simulink model "ThreePhasejojo"  (R2024a)
settings: Solver=VariableStepAuto  StartTime=0.0  StopTime=0.12  FixedStep=0.001s  MaxStep=0.00001  RelTol=1e-4
undefined symbols (not defined in the file): D1, Delta
libraries: spsVoltageMeasurementLib x19, spsCurrentMeasurementLib x12, spsPowerLib x10, spsACVoltageSourceLib x3, spsThreePhaseSeriesRLCBranchLib x3, spsGroundLib x3, spsSeriesRLCBranchLib x3, spsThreePhaseTransformerTwoWindingsLib x1, spsMutualInductanceLib x1, spspowerguiLib x1
settings Model: Creator=admin  LastModifiedBy=Asus

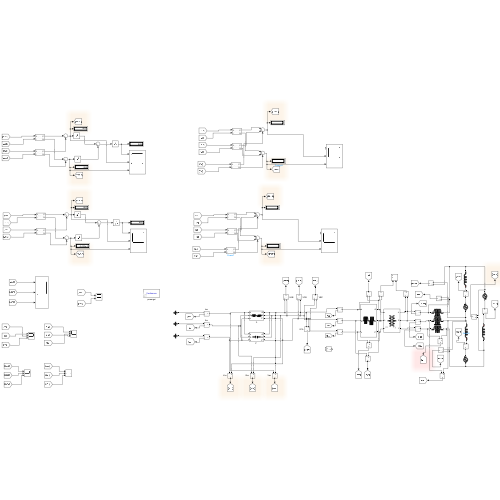
[thumbnail: Simulink's stored preview of the top-level diagram]
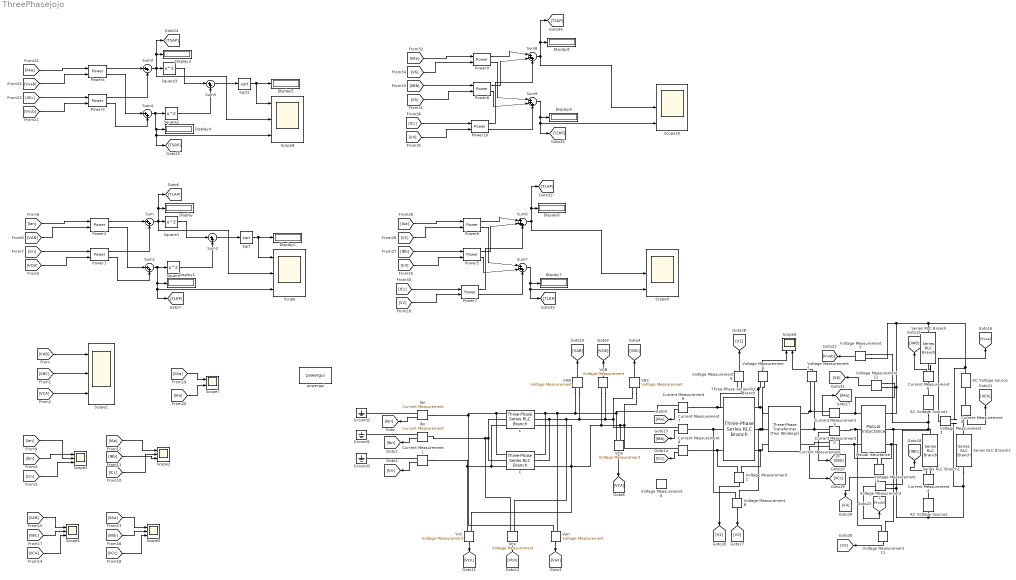
== system ThreePhasejojo ==
  " " : spsThreePhaseTransformerTwoWindingsLib/Three-Phase Transformer (Two Windings)  Winding1Connection=Yg  Winding2Connection=Delta (D1)  CoreType=Three single-phase transformers  SetSaturation=off  Hysteresis=off  DataFile='hysteresis'  SetInitialFlux=off  Measurements=None  UNITS=SI  NominalPower=[ 250e6 , 50 ]  Winding1=[380 1e-3 1e-3]  Winding2=[760 1e-3 1e-3]  Rm=1e3  Lm=1e3  L0=2.866  Saturation=[0 0;0.66653 1910.3;277.72 2419.7]  InitialFluxes=[1273.5 -1273.5 1114.3]  BreakLoop=off  DiscreteSolver=Trapezoidal iterative  DataType=on  TransfoNumber=1
  AC Voltage Source : spsACVoltageSourceLib/AC Voltage Source  Amplitude=380  Phase=-120  Frequency=50  SampleTime=0  Measurements=None  BusType=swing  Pref=10e3  Qref=0  Qmin=-inf  Qmax=+inf
  AC Voltage Source1 : spsACVoltageSourceLib/AC Voltage Source  Amplitude=380  Phase=0  Frequency=50  SampleTime=0  Measurements=None  BusType=swing  Pref=10e3  Qref=0  Qmin=-inf  Qmax=+inf
  AC Voltage Source2 : spsACVoltageSourceLib/AC Voltage Source  Amplitude=380  Phase=120  Frequency=50  SampleTime=0  Measurements=None  BusType=swing  Pref=10e3  Qref=0  Qmin=-inf  Qmax=+inf
  "C " : spsThreePhaseSeriesRLCBranchLib/Three-Phase Series RLC Branch  LConnTagsString=A|B|C  RConnTagsString=A|B|C  BranchType=C  Resistance=20  Inductance=0.1/pi  Capacitance=2e-4/pi  Measurements=None
  Current Measurement{1..10} (10 alike) : spsCurrentMeasurementLib/Current Measurement  PhasorSimulation=off  OutputType=Complex  PSBequivalent=0
  Display{,1..9} (10 alike) : Display
  Ground1 : spsGroundLib/Ground  LConnTagsString=a
  Ground2 : spsGroundLib/Ground  LConnTagsString=a
  Ground3 : spsGroundLib/Ground  LConnTagsString=a
  Ian : spsCurrentMeasurementLib/Current Measurement  PhasorSimulation=off  OutputType=Complex  PSBequivalent=0
  Ibn : spsCurrentMeasurementLib/Current Measurement  PhasorSimulation=off  OutputType=Complex  PSBequivalent=0
  L : spsThreePhaseSeriesRLCBranchLib/Three-Phase Series RLC Branch  LConnTagsString=A|B|C  RConnTagsString=A|B|C  BranchType=RL  Resistance=20  Inductance=0.1/pi  Capacitance=1e-6  Measurements=None
  Mutual Inductance : spsMutualInductanceLib/Mutual Inductance  LConnTagsString=a|b|c  RConnTagsString=A|B|C  TypeOfMutual=Two or three windings with equal mutual terms  NumberOfWindings=3  SelfImpedance1=[ 1e-3 0.02/pi ]  SelfImpedance2=[ 1e-3 0.02/pi ]  ThreeWindings=on  SelfImpedance3=[ 1e-3 0.02/pi ]  MutualImpedance=[ 0 0.01/pi ]  InductanceMatrix="[1.0 0.9  0.9 ;  0.9 1.0  0.9;  0.9 0.9 1.0 ] * 1e-3"  ResistanceMatrix="[1.0 0.9  0.9 ;  0.9 1.0  0.9;  0.9 0.9 1.0 ]"  Measurements=None
      settings: LibrarySourceBlock=sps_lib/Passives/Mutual Inductance
  Power{1..10} (10 alike) : spsPowerLib/Power  Freq=60  Vinit=[1, 0]  Iinit=[1, 0]  Ts=0
  Scope{,1..5,8..10} (9 alike) : Scope  NumInputPorts=3
  Scope6 : Scope  NumInputPorts=2
  Scope7 : Scope  NumInputPorts=2
  Series RLC Branch : spsSeriesRLCBranchLib/Series RLC Branch  LConnTagsString=__new0  RConnTagsString=__new0  BranchType=L  Resistance=1  Inductance=0.01/pi  SetiL0=off  InitialCurrent=0  Capacitance=1e-6  Setx0=off  InitialVoltage=0  Measurements=None
  Series RLC Branch1 : spsSeriesRLCBranchLib/Series RLC Branch  LConnTagsString=__new0  RConnTagsString=__new0  BranchType=L  Resistance=1  Inductance=0.01/pi  SetiL0=off  InitialCurrent=0  Capacitance=1e-6  Setx0=off  InitialVoltage=0  Measurements=None
  Series RLC Branch2 : spsSeriesRLCBranchLib/Series RLC Branch  LConnTagsString=__new0  RConnTagsString=__new0  BranchType=L  Resistance=1  Inductance=0.01/pi  SetiL0=off  InitialCurrent=0  Capacitance=1e-6  Setx0=off  InitialVoltage=0  Measurements=None
  Sqrt : Sqrt
  Sqrt1 : Sqrt
  Square{,1..3} (4 alike) : Math  Operator=square
  Sum{,1..5} (6 alike) : Sum  Inputs=|++
  Sum{6..9} (4 alike) : Sum  Inputs=|+++
  Three-Phase Series RLC Branch : spsThreePhaseSeriesRLCBranchLib/Three-Phase Series RLC Branch  LConnTagsString=A|B|C  RConnTagsString=A|B|C  BranchType=RL  Resistance=1  Inductance=0.03/pi  Capacitance=1e-6  Measurements=None
  VAB : spsVoltageMeasurementLib/Voltage Measurement  PhasorSimulation=off  OutputType=Complex  PSBequivalent=0
  VBC : spsVoltageMeasurementLib/Voltage Measurement  PhasorSimulation=off  OutputType=Complex  PSBequivalent=0
  VCA : spsVoltageMeasurementLib/Voltage Measurement  PhasorSimulation=off  OutputType=Complex  PSBequivalent=0
  VCB : spsVoltageMeasurementLib/Voltage Measurement  PhasorSimulation=off  OutputType=Complex  PSBequivalent=0
  Van : spsVoltageMeasurementLib/Voltage Measurement  PhasorSimulation=off  OutputType=Complex  PSBequivalent=0
  Vbn : spsVoltageMeasurementLib/Voltage Measurement  PhasorSimulation=off  OutputType=Complex  PSBequivalent=0
  Vcn : spsVoltageMeasurementLib/Voltage Measurement  PhasorSimulation=off  OutputType=Complex  PSBequivalent=0
  Voltage Measurement{1..12} (12 alike) : spsVoltageMeasurementLib/Voltage Measurement  PhasorSimulation=off  OutputType=Complex  PSBequivalent=0
  powergui : spspowerguiLib/powergui  Priority=1  SimulationMode=Continuous  SampleTime=50e-6  frequency=60  Iterations=50  frequencyindice=50  Pbase=100e6  ErrMax=1e-4  UnitsV=kV  UnitsW=MW  buscounter=0  FunctionMessages=off  echomessages=off  EnableUseOfTLC=off  CurrentSourceSwitches=off  DisableSnubberDevices=off  DisableRonSwitches=off  DisableVfSwitches=off  DisplayEquations=off  AutomaticDiscreteSolvers=off  SolverType=Tustin/Backward Euler (TBE)  Interpol=off  ExternalGateDelay=off  methode=off  Ts=100  x0status=blocks  SPID=on  SwTol=0  HookPort=off  NonlinearTolerance=1e-4  nMaxIteration=100  ContinueOnMaxIteration=off  RestoreLinks=warning  ResistiveCurrentMeasurement=off  Frange=[0:2:500]  Ylog=off  Xlog=on  ShowGrid=off  save=off  variable=ZData  structure=0  ZoomFFT=off  StartTime=0.0  cycles=1  DisplayStyle=1  fundamental=60  FreqAxis=off  MaxFrequency=1000  frequencyindicesteady=1  RmsSteady=1  display=off
  wires:
  Ian/1 -> [Ian]
  Ibn/1 -> [Ibn]
  Current Measurement1/1 -> [Icn]
  Van/1 -> [Van]
  Vbn/1 -> [Vbn]
  Vcn/1 -> [Vcn]
  [Ian] -> Power2/1
  [VAB] -> Power2/2
  [Icn] -> Power1/1
  [VCB] -> Power1/2
  VAB/1 -> [VAB]
  VCB/1 -> [VCB]
  VCA/1 -> [VCA]
  Power2/1 -> Sum/1
  Power1/1 -> Sum/2
  Power2/2 -> Sum1/1
  Power1/2 -> Sum1/2
  Sum/1 -> Scope/2, [TLAP], Display/1, Square1/1
  Sum1/1 -> Scope/3, [TLRP], Display1/1, Square/1
  Square1/1 -> Sum2/1
  Square/1 -> Sum2/2
  Sum2/1 -> Sqrt/1
  Sqrt/1 -> Scope/1, Display2/1
  VBC/1 -> [VBC]
  [VBC] -> Scope1/2
  [VAB] -> Scope1/1
  [VCA] -> Scope1/3
  Current Measurement9/1 -> [IAa]
  Current Measurement7/1 -> [IBb]
  Current Measurement8/1 -> [ICc]
  [Icn] -> Scope3/3
  [Ibn] -> Scope3/1
  [Ian] -> Scope3/2
  [IAa] -> Scope2/1
  [IBb] -> Scope2/3
  [ICc] -> Scope2/2
  Current Measurement5/1 -> [IICA]
  Current Measurement4/1 -> [IIBC]
  Current Measurement3/1 -> [IIAa]
  Current Measurement2/1 -> [IIBb]
  Current Measurement10/1 -> [IICc]
  [IIAB] -> Scope4/1
  [IIBC] -> Scope4/2
  [IICA] -> Scope4/3
  [IIAa] -> Scope5/1
  [IIBb] -> Scope5/2
  [IICc] -> Scope5/3
  Voltage Measurement5/1 -> Scope6/2
  Voltage Measurement4/1 -> Scope6/1
  [IIAa] -> Scope7/1
  [IAa] -> Scope7/2
  Current Measurement6/1 -> [IIAB]
  Voltage Measurement3/1 -> [Vvca]
  Voltage Measurement7/1 -> [Vvab]
  Voltage Measurement1/1 -> [Vvcb]
  [IIAa] -> Power4/1
  [IICc] -> Power3/1
  [Vvcb] -> Power3/2
  Sum5/1 -> Sqrt1/1
  Power4/1 -> Sum3/1
  Sum3/1 -> Scope8/2, [TSAP], Display3/1, Square3/1
  Sqrt1/1 -> Scope8/1, Display5/1
  Power3/2 -> Sum4/2
  [Vvab] -> Power4/2
  Square2/1 -> Sum5/2
  Square3/1 -> Sum5/1
  Sum4/1 -> Scope8/3, [TSRP], Display4/1, Square2/1
  Power4/2 -> Sum4/1
  Power3/1 -> Sum3/2
  Voltage Measurement9/1 -> [V1]
  Voltage Measurement2/1 -> [V2]
  Voltage Measurement8/1 -> [V3]
  Voltage Measurement10/1 -> [V4]
  Voltage Measurement11/1 -> [V5]
  Voltage Measurement12/1 -> [V6]
  [IAa] -> Power6/1
  [IBb] -> Power5/1
  [V3] -> Power5/2
  Power6/1 -> Sum6/1
  Sum6/1 -> Scope9/2, [T1AP], Display6/1
  Power5/2 -> Sum7/2
  [V1] -> Power6/2
  Sum7/1 -> Scope9/3, [T1RP], Display7/1
  Power6/2 -> Sum7/1
  Power5/1 -> Sum6/2
  [V2] -> Power7/2
  [ICc] -> Power7/1
  Power7/1 -> Sum6/3
  Power7/2 -> Sum7/3
  [ICc] -> Power10/1
  Power10/2 -> Sum9/3
  Power8/2 -> Sum9/2
  [V4] -> Power10/2
  Sum8/1 -> Scope10/2, [T2AP], Display8/1
  Power9/1 -> Sum8/1
  [V6] -> Power9/2
  Sum9/1 -> Scope10/3, [T2RP], Display9/1
  [V5] -> Power8/2
  Power8/1 -> Sum8/2
  Power10/1 -> Sum8/3
  [IIBb] -> Power8/1
  [IIAa] -> Power9/1
  Power9/2 -> Sum9/1
  connections:
  AC Voltage Source/LConn1 -- Mutual Inductance/RConn1 -- Voltage Measurement12/LConn1 -- Voltage Measurement7/LConn1 -- Series RLC Branch/RConn1 -- Voltage Measurement3/LConn2
  Series RLC Branch2/RConn1 -- Voltage Measurement3/LConn1 -- Voltage Measurement10/LConn1 -- Mutual Inductance/RConn3 -- Voltage Measurement1/LConn1 -- AC Voltage Source2/LConn1
  "C "/LConn1 -- Van/LConn1 -- VAB/LConn1 -- Current Measurement9/RConn1 -- VCA/LConn2 -- L/LConn1
  "C "/LConn2 -- L/LConn2 -- Vbn/LConn1 -- VAB/LConn2 -- Current Measurement7/RConn1 -- VBC/LConn1 -- VCB/LConn2
  "C "/RConn1 -- Ian/LConn1 -- Van/LConn2 -- L/RConn1
  "C "/RConn2 -- Vbn/LConn2 -- Ibn/LConn1 -- L/RConn2
  "C "/RConn3 -- Current Measurement1/LConn1 -- Vcn/LConn2 -- L/RConn3
  AC Voltage Source1/LConn1 -- Voltage Measurement7/LConn2 -- Voltage Measurement11/LConn1 -- Mutual Inductance/RConn2 -- Voltage Measurement1/LConn2 -- Series RLC Branch1/RConn1
  " "/RConn1 -- Voltage Measurement9/LConn1 -- Voltage Measurement4/LConn1 -- Three-Phase Series RLC Branch/LConn1
  Three-Phase Series RLC Branch/LConn2 -- Voltage Measurement4/LConn2 -- " "/RConn2 -- Voltage Measurement8/LConn1
  " "/RConn3 -- Voltage Measurement2/LConn1 -- Three-Phase Series RLC Branch/LConn3
  "C "/LConn3 -- VCB/LConn1 -- Current Measurement8/RConn1 -- VBC/LConn2 -- VCA/LConn1 -- Vcn/LConn1 -- L/LConn3
  Ian/RConn1 -- Ground2/LConn1
  Ibn/RConn1 -- Ground1/LConn1
  Current Measurement1/RConn1 -- Ground3/LConn1
  Current Measurement9/LConn1 -- Voltage Measurement9/LConn2 -- Three-Phase Series RLC Branch/RConn1
  Three-Phase Series RLC Branch/RConn2 -- Voltage Measurement8/LConn2 -- Current Measurement7/LConn1
  Current Measurement8/LConn1 -- Voltage Measurement2/LConn2 -- Three-Phase Series RLC Branch/RConn3
  Current Measurement6/LConn1 -- AC Voltage Source1/RConn1
  Current Measurement5/LConn1 -- AC Voltage Source/RConn1
  Current Measurement5/RConn1 -- Series RLC Branch2/LConn1
  Current Measurement4/LConn1 -- AC Voltage Source2/RConn1
  Current Measurement4/RConn1 -- Series RLC Branch1/LConn1
  Current Measurement3/LConn1 -- Voltage Measurement12/LConn2 -- Mutual Inductance/LConn1
  Current Measurement3/RConn1 -- Voltage Measurement5/LConn1 -- " "/LConn1
  Current Measurement2/RConn1 -- Voltage Measurement5/LConn2 -- " "/LConn2
  Current Measurement2/LConn1 -- Voltage Measurement11/LConn2 -- Mutual Inductance/LConn2
  Current Measurement10/LConn1 -- Voltage Measurement10/LConn2 -- Mutual Inductance/LConn3
  Current Measurement10/RConn1 -- " "/LConn3
  Current Measurement6/RConn1 -- Series RLC Branch/LConn1
